simulink model "pid_enhanced21"  (Simulink 6.0)
settings: Solver=ode45  StartTime=0.0  StopTime=30  RelTol=1e-3
undefined symbols (not defined in the file): DiscIntNeverNeededParam
settings Model: LastModifiedBy=star

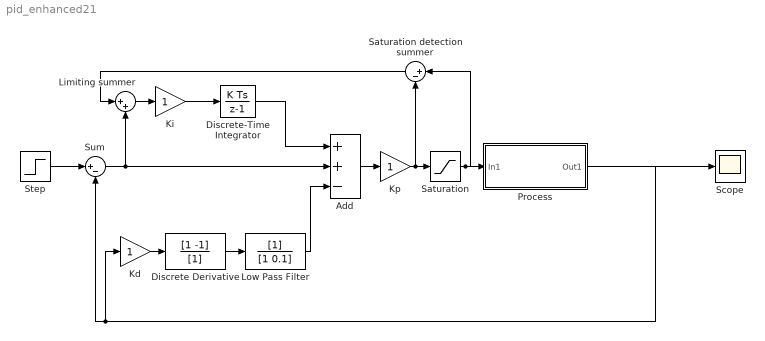
== system pid_enhanced21 ==
  Add : Sum  Inputs=++-  OutScaling=2^-10
  Discrete Derivative : DiscreteFilter  Numerator=[1 -1]  Denominator=[1]
  Discrete-Time Integrator : DiscreteIntegrator  ICPrevOutput=DiscIntNeverNeededParam  ICPrevScaledInput=DiscIntNeverNeededParam
  Kd : Gain
  Ki : Gain
  Kp : Gain
  Limiting summer : Sum  Inputs=|++
  Low Pass Filter : DiscreteFilter  Denominator=[1 0.1]
  Process : Subsystem
  Saturation : Saturate  UpperLimit=2  LowerLimit=-2
  Saturation detection summer : Sum  Orientation=left  Inputs=|+-
  Scope : Scope
  Step : Step  Time=0  SampleTime=0
  Sum : Sum  Inputs=|+-
  wires:
  Ki/1 -> Discrete-Time Integrator/1
  Add/1 -> Kp/1
  Process/1(Out1) -> Scope/1, Kd/1, Sum/2
  Kd/1 -> Discrete Derivative/1
  Step/1 -> Sum/1
  Kp/1 -> Saturation/1, Saturation detection summer/2
  Saturation/1 -> Saturation detection summer/1, Process/1(In1)
  Sum/1 -> Add/2, Limiting summer/2
  Limiting summer/1 -> Ki/1
  Discrete-Time Integrator/1 -> Add/1
  Saturation detection summer/1 -> Limiting summer/1
  Discrete Derivative/1 -> Low Pass Filter/1
  Low Pass Filter/1 -> Add/3

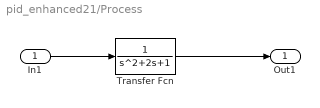
== system pid_enhanced21/Process ==
  In1 : Inport  Port=1  LatchInput=off
  Transfer Fcn : TransferFcn
  Out1 : Outport
  wires:
  In1/1 -> Transfer Fcn/1
  Transfer Fcn/1 -> Out1/1
